simulink model "Korabr"  (R2021b)
settings: Solver=VariableStepAuto  StartTime=0.0  StopTime=10.0  RelTol=1e-3
undefined symbols (not defined in the file or in its folder): drawKorabr
libraries: simulink x6
settings Model: Creator=zhour  LastModifiedBy=zhour

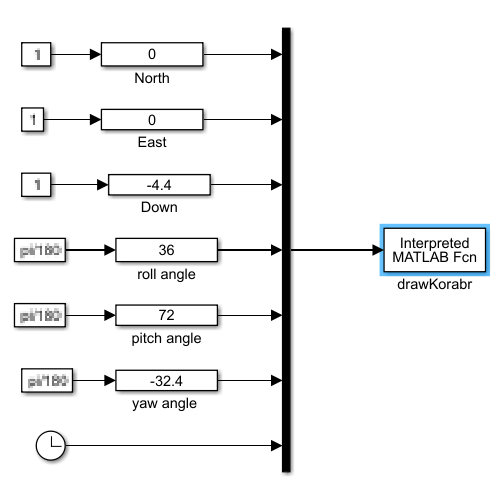
[thumbnail: Simulink's stored preview of the top-level diagram]
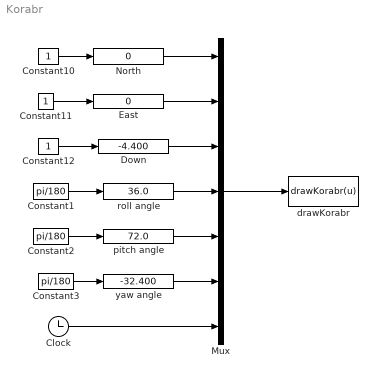
== system Korabr ==
  Clock : Clock
  Constant1 : Constant  Value=pi/180
  Constant10 : Constant
  Constant11 : Constant
  Constant12 : Constant
  Constant2 : Constant  Value=pi/180
  Constant3 : Constant  Value=pi/180
  Down : simulink/Math Operations/Slider Gain  gain=-4.400  low=-10  high=10
  East : simulink/Math Operations/Slider Gain  gain=0  low=-10  high=10
  Mux : Mux  Inputs=7
  North : simulink/Math Operations/Slider Gain  gain=0  low=-10  high=10
  drawKorabr : MATLABFcn  MATLABFcn=drawKorabr(u)  OutputDimensions=0
      mask init:
      | %太空船初始位置
      | INTs = [
      |         1 1 0;
      |         1 -1 0;
      |         -1 -1 0;
      |         -1 1 0;
      |         1 1 0;
      |         1 1 -2;
      |         1 -1 -2;
      |         1 -1 0;
      |         1 -1 -2;
      |         -1 -1 -2;
      |         -1 -1 0;
      |         -1 -1 -2;
      |         -1 1 -2;
      |         -1 1 0;
      |         -1 1 -2;
      |         1 1 -2;
      |         1 1 0;
      |         1.5 1.5 0;
      |         1.5 -1.5 0;
      |         -1.5 -1.5 0;
      |         -1 -1 0;
      |         -1.5 -1.5 0;
      |         -1.5 1.5 0;
      |         -1 1 0;
      |         -1.5 1.5 0;
      |         1.5 1.5 0;
      |         ]';
  pitch angle : simulink/Math Operations/Slider Gain  gain=72.0  low=-180  high=180
  roll angle : simulink/Math Operations/Slider Gain  gain=36.0  low=-180  high=180
  "yaw angle " : simulink/Math Operations/Slider Gain  gain=-32.400  low=-180  high=180
  wires:
  Constant10/1 -> North/1
  Constant11/1 -> East/1
  Constant12/1 -> Down/1
  Constant1/1 -> roll angle/1
  Constant2/1 -> pitch angle/1
  Constant3/1 -> "yaw angle "/1
  pitch angle/1 -> Mux/5
  "yaw angle "/1 -> Mux/6
  roll angle/1 -> Mux/4
  Down/1 -> Mux/3
  East/1 -> Mux/2
  North/1 -> Mux/1
  Mux/1 -> drawKorabr/1
  Clock/1 -> Mux/7
